simulink model "clik_transpose"  (R2022b)
settings: Solver=ode1  StartTime=0.0  StopTime=4  FixedStep=0.001  RelTol=1e-3
undefined symbols (not defined in the file or in its folder): DiscIntNeverNeededParam, q0, Tc
settings Model: Creator=Xp  LastModifiedBy=reube
settings SolverCC: AlgebraicLoopSolver=TrustRegion
settings DataIOCC: LimitDataPoints=on  SaveFormat=Array  SignalLoggingSaveFormat=ModelDataLogs  ReturnWorkspaceOutputs=off
settings OptimizationCC: ExpressionDepthLimit=2147483647  InitFltsAndDblsToZero=on  LifeSpan=inf
settings DebuggingCC: SaveWithParameterizedLinksMsg=none  UnderspecifiedInitializationDetection=Classic  MergeDetectMultiDrivingBlocksExec=none  SolverPrmCheckMsg=warning  MultiTaskDSMMsg=warning  MultiTaskCondExecSysMsg=none  FcnCallInpInsideContextMsg=warning  UnconnectedInputMsg=warning  UnconnectedOutputMsg=warning  UnconnectedLineMsg=warning  StateNameClashWarn=warning  SFUnexpectedBacktrackingDiag=warning  SFNoUnconditionalDefaultTransitionDiag=warning  SFExecutionAtInitializationDiag=none  SFMachineParentedDataDiag=warning  ArithmeticOperatorsInVariantConditions=warning
settings HardwareCC: ProdBitPerPointer=32  ProdBitPerSizeT=32  ProdBitPerPtrDiffT=32  ProdLargestAtomicFloat=None  ProdIntDivRoundTo=Undefined  ProdEndianess=Unspecified  ProdWordSize=32  ProdHWDeviceType=32-bit Generic
settings ModelReferenceCC: EnableRefExpFcnMdlSchedulingChecks=on  PropagateSignalLabelsOutOfModel=off
settings SFSimCC: CustomCodeUndefinedFunction=UseInterfaceOnly
settings RTWCC: DLArmComputeVersion=19.05
settings CodeAppCC: StateflowObjectComments=on
settings GRTTargetCC: TargetLangStandard=C89/C90 (ANSI)  CombineOutputUpdateFcns=off  GRTInterface=on
settings ConfigComp: CovMetricSettings=dw  CovSaveCumulativeToWorkspaceVar=on  CovSaveSingleToWorkspaceVar=on

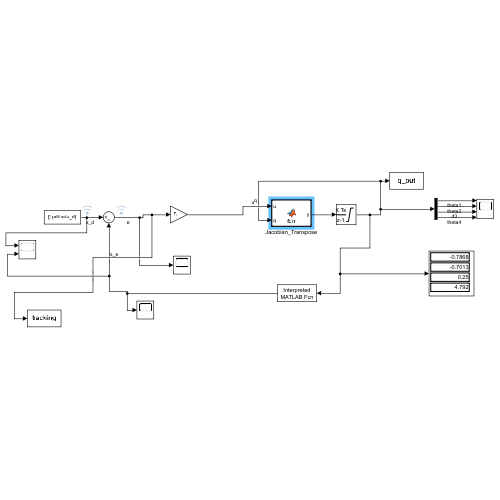
[thumbnail: Simulink's stored preview of the top-level diagram]
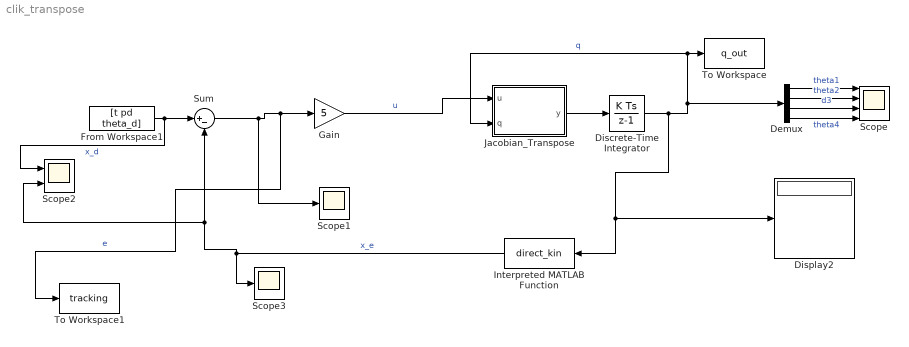
== system clik_transpose ==
  Demux : Demux
  Discrete-Time Integrator : DiscreteIntegrator  InitialCondition=q0  SampleTime=Tc  LimitOutput=on  UpperSaturationLimit=[pi/2;pi/4;1;2*pi]  LowerSaturationLimit=[-pi/2;-pi/2;0.25;-2*pi]  ICPrevOutput=DiscIntNeverNeededParam  ICPrevScaledInput=DiscIntNeverNeededParam
  Display2 : Display
  From Workspace1 : FromWorkspace  VariableName=[t pd theta_d]  SampleTime=Tc
  Gain : Gain  Gain=5
  Interpreted MATLAB Function : MATLABFcn  MATLABFcn=direct_kin  OutputDimensions=4
  Jacobian_Transpose : MATLAB Function  TreatAsAtomicUnit=on
  Scope : Scope  NumInputPorts=4
  Scope1 : Scope
  Scope2 : Scope  NumInputPorts=2
  Scope3 : Scope
  Sum : Sum  Inputs=|+-
  To Workspace : ToWorkspace  VariableName=q_out  SampleTime=Tc
  To Workspace1 : ToWorkspace  VariableName=tracking  SampleTime=Tc
  wires:
  Jacobian_Transpose/1(y) -> Discrete-Time Integrator/1
  Sum/1 -> Scope1/1, To Workspace1/1, Gain/1  "e"
  From Workspace1/1 -> Scope2/1, Sum/1  "x_d"
  Demux/3 -> Scope/3  "d3"
  Interpreted MATLAB Function/1 -> Scope2/2, Sum/2, Scope3/1  "x_e"
  Demux/4 -> Scope/4  "theta4"
  Gain/1 -> Jacobian_Transpose/1(u)  "u"
  Discrete-Time Integrator/1 -> Interpreted MATLAB Function/1, Display2/1, Demux/1, Jacobian_Transpose/2(q), To Workspace/1  "q"
  Demux/2 -> Scope/2  "theta2"
  Demux/1 -> Scope/1  "theta1"

== matlab function clik_transpose/Jacobian_Transpose ==
  data: u input; y output; q input
function y = fcn(u,q)
y=zeros(4,1);

JacT= jacobian_transpose(q)


y = JacT* u;

end
